simulink model "lab2_next_level"  (R2013a)
settings: Solver=ode1  StartTime=0.0  StopTime=300  FixedStep=0.005  RelTol=1e-3
libraries: simulink x9
Description:
  | Created by MapleSim.
settings Model: ExtModeTrigDuration=10000  Creator=MapleSim  LastModifiedBy=sunnesoft
settings SolverCC: PositivePriorityOrder=on
settings DataIOCC: SignalLoggingSaveFormat=ModelDataLogs  SignalLogging=off  DSMLogging=off
settings OptimizationCC: ExpressionDepthLimit=2147483647  InitFltsAndDblsToZero=on
settings DebuggingCC: SaveWithParameterizedLinksMsg=none  MultiTaskDSMMsg=warning  MultiTaskCondExecSysMsg=none  FcnCallInpInsideContextMsg=UseLocalSettings  StrictBusMsg=None
settings HardwareCC: TargetHWDeviceType=32-bit Generic
settings SFSimCC: SimParseCustomCode=off
settings RTWCC: SystemTargetFile=quarc_win64.tlc  TemplateMakefile=quarc_default_tmf  Description=QUARC Win64 Target  ProcessScript=quarc_win64_make_rtw_hook  IncludeERTFirstTime=on
settings STFCustomTargetCC: TargetPreCompLibLocation=C:\PROGRA~3\QUARC\lib\2011b\win64\release  GeneratePreprocessorConditionals=Disable all  GRTInterface=on  SystemTargetFile=quarc_win64.tlc
settings GRTTargetCC: TargetPreCompLibLocation=C:\PROGRA~3\QUARC\lib\2011b\win64\release  ParMdlRefBuildCompliant=off  CompOptLevelCompliant=off  ConcurrentExecutionCompliant=off  CombineOutputUpdateFcns=off  MatFileLogging=off  GRTInterface=on  ExtMode=on  ExtModeMexFile=quarc_comm

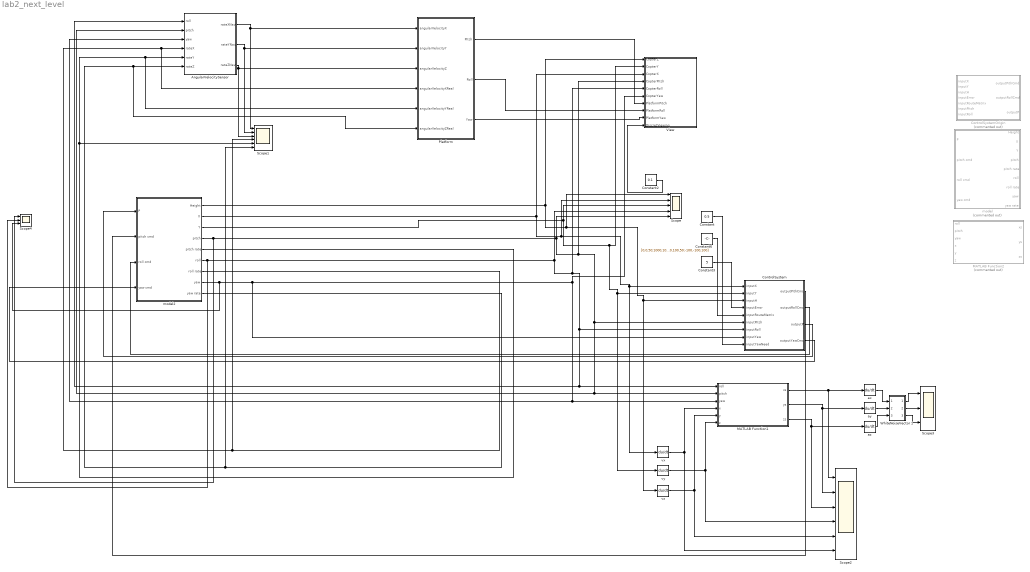
== system lab2_next_level ==
  AngularVelocitySensor : Subsystem
  Constant : Constant  Value=0.5
  Constant2 : Constant  Value=0.1
  Constant3 : Constant  Value=5
  Constant6 : Constant  Value=[0,0,50;1000,1000,50;0,20,50;100,0,50;-30,0,50;100,100,50;-100,-100,100]  VectorParams1D=off
      settings: SamplingMode=Frame based
  ControlSystem : Subsystem
  ControlSystemOrigin : Subsystem  Commented=on
  MATLAB Function1 : MATLAB Function  TreatAsAtomicUnit=on
  MATLAB Function2 : MATLAB Function  Commented=on  TreatAsAtomicUnit=on
  Platform : Subsystem
  Scope : Scope  NumInputPorts=5
      settings: TimeRange=20  YMin=0~0~0~-0.5~-1  YMax=60~450~450~1~0.5
  Scope1 : Scope  NumInputPorts=6
      settings: YMin=-1~-0.00125~-0.00125~-1~-4e-16~-2e-16  YMax=1.25~0.001~0.001~1~4e-16~5e-16
  Scope2 : Scope  NumInputPorts=6
      settings: YMin=-1.38778e-17~-7~0.5~-1~-7~-7  YMax=0.175~-1~3.5~1~-1~-1  SaveName=ScopeData2
  Scope3 : Scope  NumInputPorts=3
      settings: TimeRange=100  YMin=-45~-27.5~-3.5  YMax=15~5~4  SaveName=ScopeData3
  Scope4 : Scope  NumInputPorts=3
      settings: YMin=-0.4~-1~-2e-14  YMax=0.9~1~1e-14  SaveName=ScopeData6
  View : Subsystem
  WhiteNoiseVector 1 : Subsystem
  ax : Derivative
  ay : Derivative
  az : Derivative
  model : Subsystem  Commented=on
  model2 : Subsystem
  vx : Derivative
  vy : Derivative
  vz : Derivative
  wires:
  model2/2("X ") -> View/3(CopterX), ControlSystem/1(inputX), vx/1, Scope/2
  model2/3("Y ") -> View/2(CopterY), ControlSystem/2(inputY), vy/1, Scope/3
  model2/1("Height ") -> View/1(CopterZ), ControlSystem/3(inputH), vz/1, Scope/1
  Constant3/1 -> ControlSystem/4(inputError)
  Constant6/1 -> ControlSystem/5(inputRouteMatrix)
  ControlSystem/1(outputPithCmd) -> model2/2(pitch cmd)
  ControlSystem/2(outputRollCmd) -> model2/3(roll cmd)
  ControlSystem/3(outputP) -> model2/1(P)
  model2/4(pitch) -> Scope4/1, View/4(CopterPitch), ControlSystem/6(inputPitch), AngularVelocitySensor/2(pitch), MATLAB Function1/2(pitch), Scope/5
  model2/8(yaw) -> Scope4/3, ControlSystem/8(inputYaw), View/6(CopterYaw), AngularVelocitySensor/3(yaw), MATLAB Function1/3(yaw)
  vy/1 -> MATLAB Function1/6(z), Scope2/4
  vz/1 -> MATLAB Function1/5(y), Scope2/5
  vx/1 -> MATLAB Function1/4(x), Scope2/6
  MATLAB Function1/1(xs) -> ax/1, Scope2/1
  MATLAB Function1/2(ys) -> ay/1, Scope2/2
  MATLAB Function1/3(zs) -> az/1, Scope2/3
  WhiteNoiseVector 1/1(Out1) -> Scope3/1
  WhiteNoiseVector 1/2(Out2) -> Scope3/2
  WhiteNoiseVector 1/3(Out3) -> Scope3/3
  ay/1 -> WhiteNoiseVector 1/2(In2)
  ax/1 -> WhiteNoiseVector 1/1(In1)
  az/1 -> WhiteNoiseVector 1/3(In3)
  Constant2/1 -> View/10(DiscretViewing)
  model2/5(pitch rate) -> Platform/5(angularVelocityYReal), AngularVelocitySensor/5(rateY), Scope1/5
  model2/9(yaw rate) -> Platform/6(angularVelocityZReal), AngularVelocitySensor/6(rateZ), Scope1/6
  model2/7(roll rate) -> Platform/4(angularVelocityXReal), AngularVelocitySensor/4(rateX), Scope1/4
  AngularVelocitySensor/1(rateXNav) -> Scope1/1, Platform/1(angularVelocityX)
  AngularVelocitySensor/2(rateYNav) -> Platform/2(angularVelocityY), Scope1/2
  AngularVelocitySensor/3(rateZNav) -> Platform/3(angularVelocityZ), Scope1/3
  model2/6(roll) -> Scope4/2, View/5(CopterRoll), ControlSystem/7(inputRoll), AngularVelocitySensor/1(roll), MATLAB Function1/1(roll), Scope/4
  ControlSystem/4(outputYawCmd) -> model2/4(yaw cmd)
  Constant/1 -> ControlSystem/9(inputYawNeed)
  Platform/1(Pitch) -> View/7(PlatformPitch)
  Platform/2(Roll) -> View/8(PlatformRoll)
  Platform/3(Yaw) -> View/9(PlatformYaw)

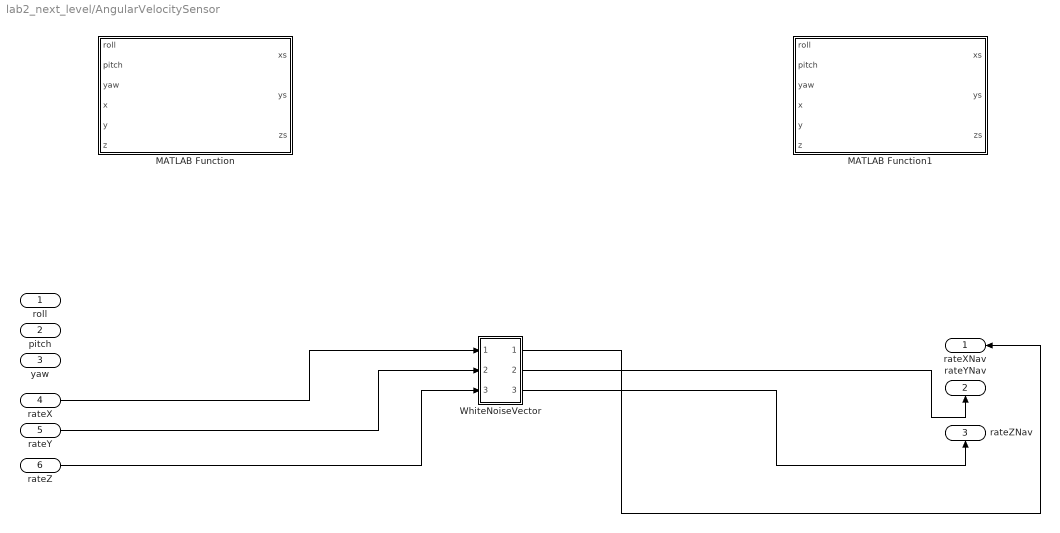
== system lab2_next_level/AngularVelocitySensor ==
  roll : Inport
  pitch : Inport  Port=2
  yaw : Inport  Port=3
  rateX : Inport  Port=4
  rateY : Inport  Port=5
  rateZ : Inport  Port=6
  MATLAB Function : MATLAB Function  TreatAsAtomicUnit=on
  MATLAB Function1 : MATLAB Function  TreatAsAtomicUnit=on
  "WhiteNoiseVector " : Subsystem
  rateXNav : Outport
  rateYNav : Outport  Port=2
  rateZNav : Outport  Port=3
  wires:
  rateX/1 -> "WhiteNoiseVector "/1(In1)
  rateY/1 -> "WhiteNoiseVector "/2(In2)
  rateZ/1 -> "WhiteNoiseVector "/3(In3)
  "WhiteNoiseVector "/1(Out1) -> rateXNav/1
  "WhiteNoiseVector "/2(Out2) -> rateYNav/1
  "WhiteNoiseVector "/3(Out3) -> rateZNav/1

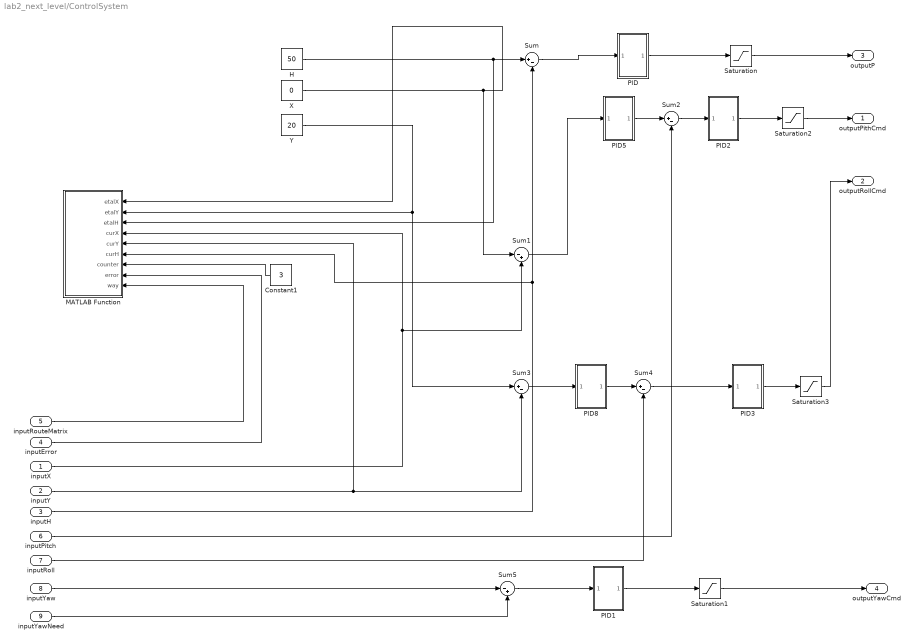
== system lab2_next_level/ControlSystem ==
  inputX : Inport
  inputY : Inport  Port=2
  inputH : Inport  Port=3
  inputError : Inport  Port=4
  inputRouteMatrix : Inport  Port=5
  inputPitch : Inport  Port=6
  inputRoll : Inport  Port=7
  inputYaw : Inport  Port=8
  inputYawNeed : Inport  Port=9
  Constant1 : Constant  InitFcn=|  Value=3
      | coder.extrinsic('set_param');                                    
      | set_param('lab2_next_level/ControlSystem/Constant1','Value','0');
  H : Constant  InitFcn=|  Value=50
      | coder.extrinsic('set_param');                            
      | set_param('lab2_next_level/ControlSystem/H','Value','0');
  MATLAB Function : MATLAB Function  TreatAsAtomicUnit=on
  PID : Subsystem
  PID1 : Subsystem
  PID2 : Subsystem
  PID3 : Subsystem
  PID5 : Subsystem
  PID8 : Subsystem
  Saturation : Saturate  UpperLimit=0.1  LowerLimit=0
  Saturation1 : Saturate  UpperLimit=0.1  LowerLimit=-0.1
  Saturation2 : Saturate  UpperLimit=0.1  LowerLimit=-0.1
  Saturation3 : Saturate  UpperLimit=0.1  LowerLimit=-0.1
  Sum{,2..4} (4 alike) : Sum  Inputs=|+-
  Sum1 : Sum  Inputs=|-+
  Sum5 : Sum  Inputs=|-+
  X : Constant  InitFcn=|  Value=0
      | coder.extrinsic('set_param');                            
      | set_param('lab2_next_level/ControlSystem/X','Value','0');
  Y : Constant  InitFcn=|  Value=20
      | coder.extrinsic('set_param');                            
      | set_param('lab2_next_level/ControlSystem/Y','Value','0');
  outputPithCmd : Outport
  outputRollCmd : Outport  Port=2
  outputP : Outport  Port=3
  outputYawCmd : Outport  Port=4
  wires:
  Saturation2/1 -> outputPithCmd/1
  PID3/1(Out1) -> Saturation3/1
  inputX/1 -> Sum1/2, MATLAB Function/4(curX)
  Saturation3/1 -> outputRollCmd/1
  PID/1(Out1) -> Saturation/1
  Saturation/1 -> outputP/1
  Constant1/1 -> MATLAB Function/7(counter)
  inputPitch/1 -> Sum2/2
  H/1 -> Sum/1, MATLAB Function/3(etalH)
  inputRouteMatrix/1 -> MATLAB Function/9(way)
  inputRoll/1 -> Sum4/2
  Sum3/1 -> PID8/1(In1)
  X/1 -> Sum1/1, MATLAB Function/1(etalX)
  Y/1 -> Sum3/1, MATLAB Function/2(etalY)
  inputError/1 -> MATLAB Function/8(error)
  inputY/1 -> Sum3/2, MATLAB Function/5(curY)
  Sum/1 -> PID/1(In1)
  inputH/1 -> MATLAB Function/6(curH), Sum/2
  PID2/1(Out1) -> Saturation2/1
  Sum1/1 -> PID5/1(In1)
  Sum2/1 -> PID2/1(In1)
  Sum4/1 -> PID3/1(In1)
  PID5/1(Out1) -> Sum2/1
  PID8/1(Out1) -> Sum4/1
  Saturation1/1 -> outputYawCmd/1
  PID1/1(Out1) -> Saturation1/1
  inputYaw/1 -> Sum5/1
  inputYawNeed/1 -> Sum5/2
  Sum5/1 -> PID1/1(In1)

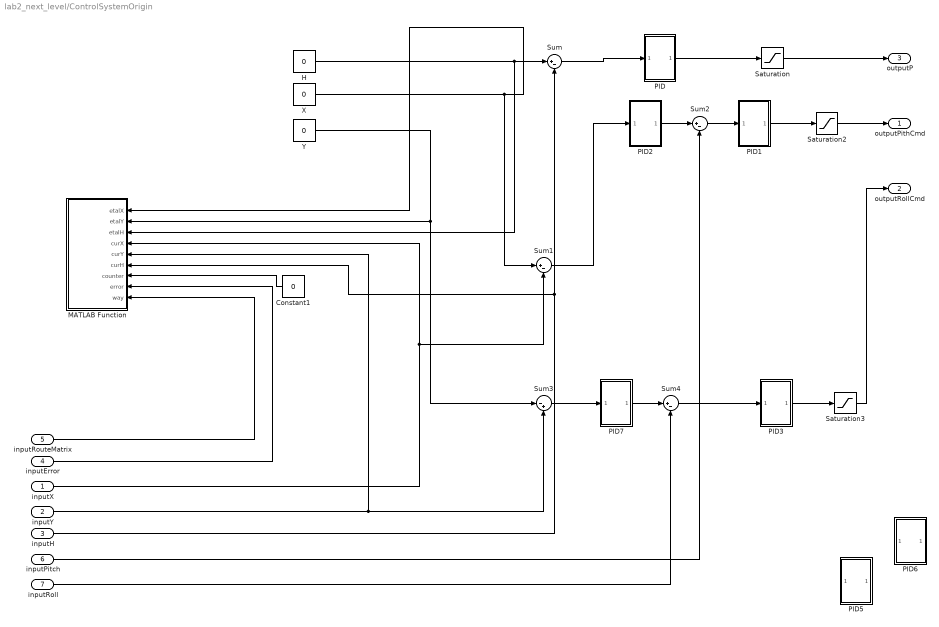
== system lab2_next_level/ControlSystemOrigin ==
  inputX : Inport
  inputY : Inport  Port=2
  inputH : Inport  Port=3
  inputError : Inport  Port=4
  inputRouteMatrix : Inport  Port=5
  inputPitch : Inport  Port=6
  inputRoll : Inport  Port=7
  Constant1 : Constant  InitFcn=|  Value=0
      | coder.extrinsic('set_param');                                    
      | set_param('lab2_next_level/ControlSystem/Constant1','Value','0');
  H : Constant  InitFcn=|  Value=0
      | coder.extrinsic('set_param');                            
      | set_param('lab2_next_level/ControlSystem/H','Value','0');
  MATLAB Function : MATLAB Function  TreatAsAtomicUnit=on
  PID : Subsystem
  PID1 : Subsystem
  PID2 : Subsystem
  PID3 : Subsystem
  PID5 : Subsystem
  PID6 : Subsystem
  PID7 : Subsystem
  Saturation : Saturate  UpperLimit=0.1  LowerLimit=0
  Saturation2 : Saturate  UpperLimit=0.1  LowerLimit=-0.1
  Saturation3 : Saturate  UpperLimit=0.01  LowerLimit=-0.01
  Sum{,1..2,4} (4 alike) : Sum  Inputs=|+-
  Sum3 : Sum  Inputs=|-+
  X : Constant  InitFcn=|  Value=0
      | coder.extrinsic('set_param');                            
      | set_param('lab2_next_level/ControlSystem/X','Value','0');
  Y : Constant  InitFcn=|  Value=0
      | coder.extrinsic('set_param');                            
      | set_param('lab2_next_level/ControlSystem/Y','Value','0');
  outputPithCmd : Outport
  outputRollCmd : Outport  Port=2
  outputP : Outport  Port=3
  wires:
  Saturation2/1 -> outputPithCmd/1
  PID3/1(Out1) -> Saturation3/1
  inputX/1 -> Sum1/2, MATLAB Function/4(curX)
  Saturation3/1 -> outputRollCmd/1
  PID/1(Out1) -> Saturation/1
  Saturation/1 -> outputP/1
  Constant1/1 -> MATLAB Function/7(counter)
  inputPitch/1 -> Sum2/2
  H/1 -> Sum/1, MATLAB Function/3(etalH)
  inputRouteMatrix/1 -> MATLAB Function/9(way)
  inputRoll/1 -> Sum4/2
  Sum3/1 -> PID7/1(In1)
  X/1 -> Sum1/1, MATLAB Function/1(etalX)
  Y/1 -> Sum3/1, MATLAB Function/2(etalY)
  inputError/1 -> MATLAB Function/8(error)
  inputY/1 -> Sum3/2, MATLAB Function/5(curY)
  Sum/1 -> PID/1(In1)
  inputH/1 -> MATLAB Function/6(curH), Sum/2
  PID1/1(Out1) -> Saturation2/1
  Sum1/1 -> PID2/1(In1)
  Sum2/1 -> PID1/1(In1)
  Sum4/1 -> PID3/1(In1)
  PID2/1(Out1) -> Sum2/1
  PID7/1(Out1) -> Sum4/1

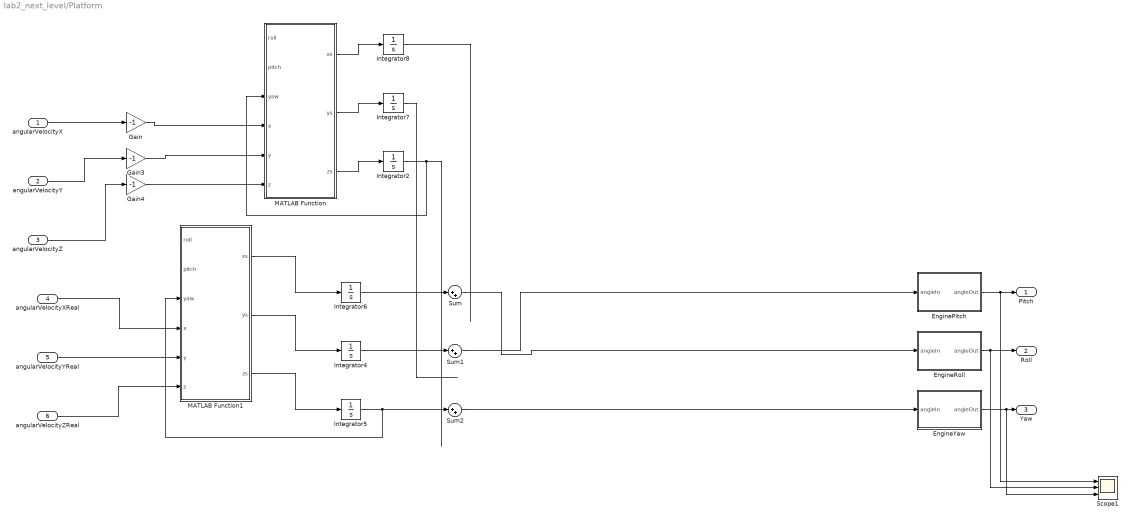
== system lab2_next_level/Platform ==
  angularVelocityX : Inport
  angularVelocityY : Inport  Port=2
  angularVelocityZ : Inport  Port=3
  angularVelocityXReal : Inport  Port=4
  angularVelocityYReal : Inport  Port=5
  angularVelocityZReal : Inport  Port=6
  EnginePitch : Subsystem
  EngineRoll : Subsystem
  EngineYaw : Subsystem
  Gain : Gain  Gain=-1
  Gain3 : Gain  Gain=-1
  Gain4 : Gain  Gain=-1
  Integrator{2,4..8} (6 alike) : Integrator  LimitOutput=on  UpperSaturationLimit=1  LowerSaturationLimit=-1
  MATLAB Function : MATLAB Function  TreatAsAtomicUnit=on
  MATLAB Function1 : MATLAB Function  TreatAsAtomicUnit=on
  Scope1 : Scope  NumInputPorts=3
      settings: TimeRange=10  YMin=-0.002~-0.0007~-0.0025  YMax=0.004~0.0003~0.0025  SaveName=ScopeData4
  Sum : Sum  Inputs=|++
  Sum1 : Sum  Inputs=|++
  Sum2 : Sum  Inputs=|++
  Pitch : Outport
  Roll : Outport  Port=2
  Yaw : Outport  Port=3
  wires:
  Integrator7/1 -> ?
  Integrator2/1 -> MATLAB Function/3(yaw)
  MATLAB Function/3(zs) -> Integrator2/1
  Integrator8/1 -> ?
  MATLAB Function/1(xs) -> Integrator8/1
  MATLAB Function/2(ys) -> Integrator7/1
  Gain/1 -> MATLAB Function/4(x)
  Gain3/1 -> MATLAB Function/5(y)
  Gain4/1 -> MATLAB Function/6(z)
  Integrator6/1 -> Sum/1
  Integrator4/1 -> Sum1/1
  Integrator5/1 -> MATLAB Function1/3(yaw), Sum2/1
  Sum2/1 -> EngineYaw/1(angleIn)
  Sum/1 -> EngineRoll/1(angleIn)
  Sum1/1 -> EnginePitch/1(angleIn)
  MATLAB Function1/1(xs) -> Integrator6/1
  MATLAB Function1/2(ys) -> Integrator4/1
  MATLAB Function1/3(zs) -> Integrator5/1
  angularVelocityX/1 -> Gain/1
  angularVelocityY/1 -> Gain3/1
  angularVelocityZ/1 -> Gain4/1
  angularVelocityXReal/1 -> MATLAB Function1/4(x)
  angularVelocityYReal/1 -> MATLAB Function1/5(y)
  angularVelocityZReal/1 -> MATLAB Function1/6(z)
  EngineRoll/1(angleOut) -> Scope1/2, Roll/1
  EngineYaw/1(angleOut) -> Scope1/3, Yaw/1
  EnginePitch/1(angleOut) -> Scope1/1, Pitch/1

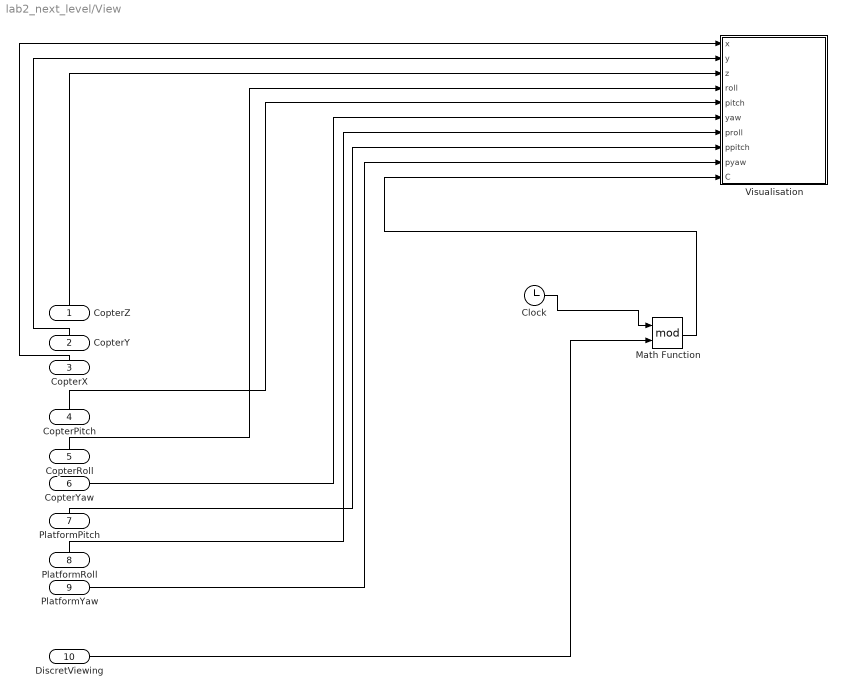
== system lab2_next_level/View ==
  CopterZ : Inport
  CopterY : Inport  Port=2
  CopterX : Inport  Port=3
  CopterPitch : Inport  Port=4
  CopterRoll : Inport  Port=5
  CopterYaw : Inport  Port=6
  PlatformPitch : Inport  Port=7
  PlatformRoll : Inport  Port=8
  PlatformYaw : Inport  Port=9
  DiscretViewing : Inport  Port=10
  Clock : Clock
  Math Function : Math  Operator=mod  SaturateOnIntegerOverflow=on
  Visualisation : MATLAB Function  TreatAsAtomicUnit=on
  wires:
  DiscretViewing/1 -> Math Function/2
  Math Function/1 -> Visualisation/10(C)
  Clock/1 -> Math Function/1
  CopterYaw/1 -> Visualisation/6(yaw)
  CopterZ/1 -> Visualisation/3(z)
  CopterPitch/1 -> Visualisation/5(pitch)
  CopterRoll/1 -> Visualisation/4(roll)
  CopterY/1 -> Visualisation/2(y)
  CopterX/1 -> Visualisation/1(x)
  PlatformYaw/1 -> Visualisation/9(pyaw)
  PlatformPitch/1 -> Visualisation/8(ppitch)
  PlatformRoll/1 -> Visualisation/7(proll)

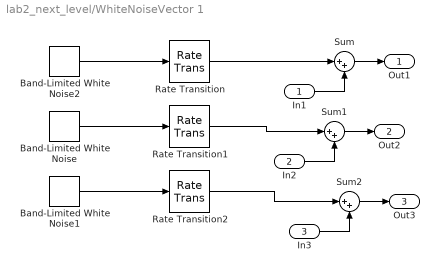
== system lab2_next_level/WhiteNoiseVector 1 ==
  In1 : Inport
  In2 : Inport  Port=2
  In3 : Inport  Port=3
  Band-Limited White Noise : simulink/Sources/Band-Limited White Noise  Cov=[0.1]  Ts=0.1  seed=[23341]
  Band-Limited White Noise1 : simulink/Sources/Band-Limited White Noise  Cov=[0.1]  Ts=0.1  seed=[23341]
  Band-Limited White Noise2 : simulink/Sources/Band-Limited White Noise  Cov=[0.1]  Ts=0.1  seed=[23341]
  Rate Transition : RateTransition
  Rate Transition1 : RateTransition
  Rate Transition2 : RateTransition
  Sum : Sum  Inputs=|++
  Sum1 : Sum  Inputs=|++
  Sum2 : Sum  Inputs=|++
  Out1 : Outport
  Out2 : Outport  Port=2
  Out3 : Outport  Port=3
  wires:
  Band-Limited White Noise2/1 -> Rate Transition/1
  Band-Limited White Noise/1 -> Rate Transition1/1
  Sum/1 -> Out1/1
  Band-Limited White Noise1/1 -> Rate Transition2/1
  Rate Transition/1 -> Sum/1
  In1/1 -> Sum/2
  Sum1/1 -> Out2/1
  Rate Transition1/1 -> Sum1/1
  In2/1 -> Sum1/2
  Sum2/1 -> Out3/1
  Rate Transition2/1 -> Sum2/1
  In3/1 -> Sum2/2

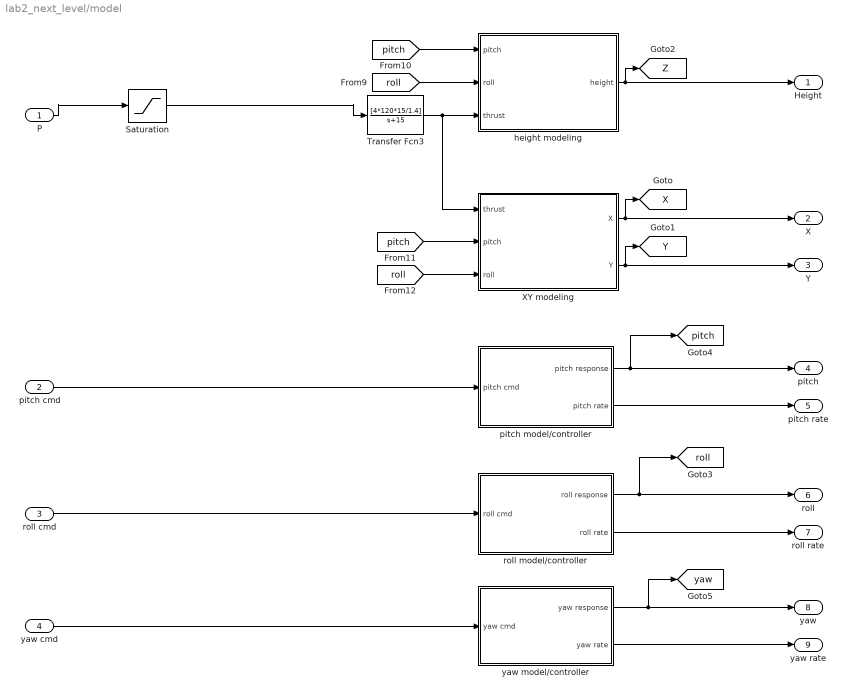
== system lab2_next_level/model ==
  P : Inport
  pitch cmd : Inport  Port=2
  roll cmd : Inport  Port=3
  yaw cmd : Inport  Port=4
  Saturation : Saturate  UpperLimit=0.1  LowerLimit=0
  Transfer Fcn3 : TransferFcn  Numerator=[4*120*15/1.4]  Denominator=[1 15]
  XY modeling : Subsystem
  height modeling : Subsystem
  pitch model/controller : Subsystem
  roll model/controller : Subsystem
  yaw model/controller : Subsystem
  "Height " : Outport
  "X " : Outport  Port=2
  "Y " : Outport  Port=3
  pitch : Outport  Port=4
  pitch rate : Outport  Port=5
  roll : Outport  Port=6
  roll rate : Outport  Port=7
  yaw : Outport  Port=8
  yaw rate : Outport  Port=9
  tag scope: X=global, Y=global, Z=global, pitch=global, roll=global, yaw=global
  wires:
  yaw cmd/1 -> yaw model/controller/1(yaw cmd)
  roll cmd/1 -> roll model/controller/1(roll cmd)
  pitch cmd/1 -> pitch model/controller/1(pitch cmd)
  P/1 -> Saturation/1
  yaw model/controller/2(yaw rate) -> yaw rate/1
  roll model/controller/2(roll rate) -> roll rate/1
  pitch model/controller/2(pitch rate) -> pitch rate/1
  XY modeling/2(Y) -> "Y "/1, [Y]
  XY modeling/1(X) -> "X "/1, [X]
  [roll] -> XY modeling/3(roll)
  [pitch] -> XY modeling/2(pitch)
  Transfer Fcn3/1 -> XY modeling/1(thrust), height modeling/3(thrust)
  [roll] -> height modeling/2(roll)
  [pitch] -> height modeling/1(pitch)
  height modeling/1(height) -> "Height "/1, [Z]
  yaw model/controller/1(yaw response) -> yaw/1, [yaw]
  roll model/controller/1(roll response) -> roll/1, [roll]
  pitch model/controller/1(pitch response) -> [pitch], pitch/1
  Saturation/1 -> Transfer Fcn3/1

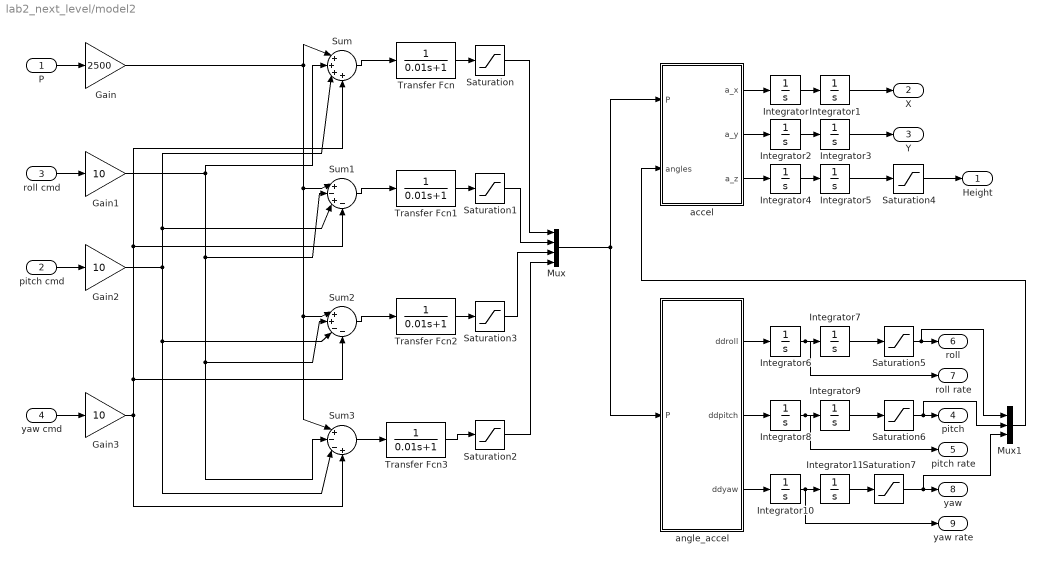
== system lab2_next_level/model2 ==
  P : Inport
  pitch cmd : Inport  Port=2
  roll cmd : Inport  Port=3
  yaw cmd : Inport  Port=4
  Gain : Gain  Gain=2500
  Gain1 : Gain  Gain=10
  Gain2 : Gain  Gain=10
  Gain3 : Gain  Gain=10
  Integrator{,1..5,10..11} (8 alike) : Integrator
  Integrator{6..9} (4 alike) : Integrator  LimitOutput=on  UpperSaturationLimit=1  LowerSaturationLimit=-1
  Mux : Mux
  Mux1 : Mux  Inputs=3
  Saturation{,1..3} (4 alike) : Saturate  UpperLimit=500  LowerLimit=0
  Saturation4 : Saturate  UpperLimit=100000000  LowerLimit=0
  Saturation5 : Saturate  UpperLimit=1  LowerLimit=-1
  Saturation6 : Saturate  UpperLimit=1  LowerLimit=-1
  Saturation7 : Saturate  UpperLimit=1  LowerLimit=-1
  Sum : Sum  Inputs=|++++
  Sum1 : Sum  Inputs=|+-+-
  Sum2 : Sum  Inputs=|++--
  Sum3 : Sum  Inputs=|+--+
  Transfer Fcn{,1..3} (4 alike) : TransferFcn  Denominator=[0.01 1]
  accel : MATLAB Function  TreatAsAtomicUnit=on
  angle_accel : MATLAB Function  TreatAsAtomicUnit=on
  "Height " : Outport
  "X " : Outport  Port=2
  "Y " : Outport  Port=3
  pitch : Outport  Port=4
  pitch rate : Outport  Port=5
  roll : Outport  Port=6
  roll rate : Outport  Port=7
  yaw : Outport  Port=8
  yaw rate : Outport  Port=9
  wires:
  P/1 -> Gain/1
  Gain/1 -> Sum1/1, Sum3/1, Sum2/1, Sum/1
  Sum/1 -> Transfer Fcn/1
  Sum1/1 -> Transfer Fcn1/1
  Sum2/1 -> Transfer Fcn2/1
  Sum3/1 -> Transfer Fcn3/1
  Transfer Fcn/1 -> Saturation/1
  Mux/1 -> accel/1(P), angle_accel/1(P)
  Integrator/1 -> Integrator1/1
  Integrator2/1 -> Integrator3/1
  Integrator4/1 -> Integrator5/1
  accel/1(a_x) -> Integrator/1
  accel/2(a_y) -> Integrator2/1
  accel/3(a_z) -> Integrator4/1
  Integrator1/1 -> "X "/1
  Integrator3/1 -> "Y "/1
  Integrator5/1 -> Saturation4/1
  angle_accel/1(ddroll) -> Integrator6/1
  Integrator6/1 -> roll rate/1, Integrator7/1
  angle_accel/3(ddyaw) -> Integrator10/1
  angle_accel/2(ddpitch) -> Integrator8/1
  Integrator8/1 -> pitch rate/1, Integrator9/1
  Integrator10/1 -> yaw rate/1, Integrator11/1
  Integrator7/1 -> Saturation5/1
  Integrator9/1 -> Saturation6/1
  Integrator11/1 -> Saturation7/1
  Saturation/1 -> Mux/1
  Transfer Fcn1/1 -> Saturation1/1
  Saturation1/1 -> Mux/2
  Saturation2/1 -> Mux/4
  Transfer Fcn2/1 -> Saturation3/1
  Saturation3/1 -> Mux/3
  yaw cmd/1 -> Gain3/1
  Saturation4/1 -> "Height "/1
  Saturation5/1 -> Mux1/1, roll/1
  Saturation6/1 -> Mux1/2, pitch/1
  roll cmd/1 -> Gain1/1
  pitch cmd/1 -> Gain2/1
  Saturation7/1 -> Mux1/3, yaw/1
  Mux1/1 -> accel/2(angles)
  Gain1/1 -> Sum2/2, Sum3/2, Sum1/2, Sum/2
  Gain2/1 -> Sum1/3, Sum/3, Sum2/3, Sum3/3
  Gain3/1 -> Sum2/4, Sum1/4, Sum/4, Sum3/4
  Transfer Fcn3/1 -> Saturation2/1

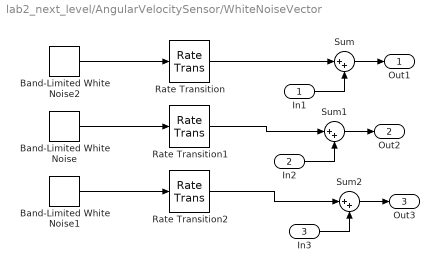
== system lab2_next_level/AngularVelocitySensor/WhiteNoiseVector  ==
  In1 : Inport
  In2 : Inport  Port=2
  In3 : Inport  Port=3
  Band-Limited White Noise : simulink/Sources/Band-Limited White Noise  Cov=[1e-8]  Ts=0.1  seed=[23341]
  Band-Limited White Noise1 : simulink/Sources/Band-Limited White Noise  Cov=[1e-8]  Ts=0.1  seed=[23341]
  Band-Limited White Noise2 : simulink/Sources/Band-Limited White Noise  Cov=[1e-8]  Ts=0.1  seed=[23341]
  Rate Transition : RateTransition
  Rate Transition1 : RateTransition
  Rate Transition2 : RateTransition
  Sum : Sum  Inputs=|++
  Sum1 : Sum  Inputs=|++
  Sum2 : Sum  Inputs=|++
  Out1 : Outport
  Out2 : Outport  Port=2
  Out3 : Outport  Port=3
  wires:
  Band-Limited White Noise2/1 -> Rate Transition/1
  Band-Limited White Noise/1 -> Rate Transition1/1
  Sum/1 -> Out1/1
  Band-Limited White Noise1/1 -> Rate Transition2/1
  Rate Transition/1 -> Sum/1
  In1/1 -> Sum/2
  Sum1/1 -> Out2/1
  Rate Transition1/1 -> Sum1/1
  In2/1 -> Sum1/2
  Sum2/1 -> Out3/1
  Rate Transition2/1 -> Sum2/1
  In3/1 -> Sum2/2

== system lab2_next_level/ControlSystem/PID ==
  In1 : Inport
  Derivative : Derivative
  Gain : Gain  Gain=0.007
  Gain1 : Gain  Gain=0.0006
  Gain2 : Gain  Gain=0.02
  Gain3 : Gain
  Integrator : Integrator
  Sum1 : Sum  Inputs=|+++
  Out1 : Outport
  wires:
  Gain1/1 -> Integrator/1
  Gain3/1 -> Sum1/1
  Integrator/1 -> Sum1/2
  Gain/1 -> Gain3/1
  In1/1 -> Gain1/1, Gain/1, Gain2/1
  Derivative/1 -> Sum1/3
  Gain2/1 -> Derivative/1
  Sum1/1 -> Out1/1

== system lab2_next_level/ControlSystem/PID1 ==
  In1 : Inport
  Derivative : Derivative
  Gain : Gain  Gain=0.012
  Gain1 : Gain  Gain=0.00048
  Gain2 : Gain  Gain=0.075
  Gain3 : Gain
  Integrator : Integrator
  Sum1 : Sum  Inputs=|+++
  Out1 : Outport
  wires:
  Gain1/1 -> Integrator/1
  Gain3/1 -> Sum1/1
  Integrator/1 -> Sum1/2
  Gain/1 -> Gain3/1
  In1/1 -> Gain1/1, Gain/1, Gain2/1
  Derivative/1 -> Sum1/3
  Gain2/1 -> Derivative/1
  Sum1/1 -> Out1/1

== system lab2_next_level/ControlSystem/PID2 ==
  In1 : Inport
  Derivative : Derivative
  Gain : Gain  Gain=0.02
  Gain1 : Gain  Gain=1e-9
  Gain2 : Gain  Gain=0.2
  Gain3 : Gain
  Integrator : Integrator
  Sum1 : Sum  Inputs=|+++
  Out1 : Outport
  wires:
  Gain1/1 -> Integrator/1
  Gain3/1 -> Sum1/1
  Integrator/1 -> Sum1/2
  Gain/1 -> Gain3/1
  In1/1 -> Gain1/1, Gain/1, Gain2/1
  Derivative/1 -> Sum1/3
  Gain2/1 -> Derivative/1
  Sum1/1 -> Out1/1

== system lab2_next_level/ControlSystem/PID3 ==
  In1 : Inport
  Derivative : Derivative
  Gain : Gain  Gain=0.02
  Gain1 : Gain  Gain=1e-9
  Gain2 : Gain  Gain=0.2
  Gain3 : Gain
  Integrator : Integrator
  Sum1 : Sum  Inputs=|+++
  Out1 : Outport
  wires:
  Gain1/1 -> Integrator/1
  Gain3/1 -> Sum1/1
  Integrator/1 -> Sum1/2
  Gain/1 -> Gain3/1
  In1/1 -> Gain1/1, Gain/1, Gain2/1
  Derivative/1 -> Sum1/3
  Gain2/1 -> Derivative/1
  Sum1/1 -> Out1/1

== system lab2_next_level/ControlSystem/PID5 ==
  In1 : Inport
  Derivative : Derivative
  Gain : Gain  Gain=0.1
  Gain1 : Gain  Gain=1e-9
  Gain2 : Gain  Gain=0.35
  Gain3 : Gain
  Integrator : Integrator
  Sum1 : Sum  Inputs=|+++
  Out1 : Outport
  wires:
  Gain1/1 -> Integrator/1
  Gain3/1 -> Sum1/1
  Integrator/1 -> Sum1/2
  Gain/1 -> Gain3/1
  In1/1 -> Gain1/1, Gain/1, Gain2/1
  Derivative/1 -> Sum1/3
  Gain2/1 -> Derivative/1
  Sum1/1 -> Out1/1

== system lab2_next_level/ControlSystem/PID8 ==
  In1 : Inport
  Derivative : Derivative
  Gain : Gain  Gain=0.1
  Gain1 : Gain  Gain=1e-9
  Gain2 : Gain  Gain=0.35
  Gain3 : Gain
  Integrator : Integrator
  Sum1 : Sum  Inputs=|+++
  Out1 : Outport
  wires:
  Gain1/1 -> Integrator/1
  Gain3/1 -> Sum1/1
  Integrator/1 -> Sum1/2
  Gain/1 -> Gain3/1
  In1/1 -> Gain1/1, Gain/1, Gain2/1
  Derivative/1 -> Sum1/3
  Gain2/1 -> Derivative/1
  Sum1/1 -> Out1/1

== system lab2_next_level/ControlSystemOrigin/PID ==
  In1 : Inport
  Derivative : Derivative
  Gain : Gain  Gain=0.006
  Gain1 : Gain  Gain=3.831578947e-04
  Gain2 : Gain  Gain=0.0361325
  Gain3 : Gain
  Integrator : Integrator
  Sum1 : Sum  Inputs=|+++
  Out1 : Outport
  wires:
  Gain1/1 -> Integrator/1
  Gain3/1 -> Sum1/1
  Integrator/1 -> Sum1/2
  Gain/1 -> Gain3/1
  In1/1 -> Gain1/1, Gain/1, Gain2/1
  Derivative/1 -> Sum1/3
  Gain2/1 -> Derivative/1
  Sum1/1 -> Out1/1

== system lab2_next_level/ControlSystemOrigin/PID1 ==
  In1 : Inport
  Derivative : Derivative
  Gain : Gain  Gain=6e-03
  Gain1 : Gain  Gain=6e-9
  Gain2 : Gain  Gain=0.0255
  Gain3 : Gain
  Integrator : Integrator
  Sum1 : Sum  Inputs=|+++
  Out1 : Outport
  wires:
  Gain1/1 -> Integrator/1
  Gain3/1 -> Sum1/1
  Integrator/1 -> Sum1/2
  Gain/1 -> Gain3/1
  In1/1 -> Gain1/1, Gain/1, Gain2/1
  Derivative/1 -> Sum1/3
  Gain2/1 -> Derivative/1
  Sum1/1 -> Out1/1

== system lab2_next_level/ControlSystemOrigin/PID2 ==
  In1 : Inport
  Derivative : Derivative
  Gain : Gain  Gain=0.010
  Gain1 : Gain  Gain=7.058823529e-09
  Gain2 : Gain  Gain=0.141875
  Gain3 : Gain
  Integrator : Integrator
  Sum1 : Sum  Inputs=|+++
  Out1 : Outport
  wires:
  Gain1/1 -> Integrator/1
  Gain3/1 -> Sum1/1
  Integrator/1 -> Sum1/2
  Gain/1 -> Gain3/1
  In1/1 -> Gain1/1, Gain/1, Gain2/1
  Derivative/1 -> Sum1/3
  Gain2/1 -> Derivative/1
  Sum1/1 -> Out1/1

== system lab2_next_level/ControlSystemOrigin/PID3 ==
  In1 : Inport
  Derivative : Derivative
  Gain : Gain  Gain=5e-03
  Gain1 : Gain  Gain=6e-9
  Gain2 : Gain  Gain=0.035
  Gain3 : Gain
  Integrator : Integrator
  Sum1 : Sum  Inputs=|+++
  Out1 : Outport
  wires:
  Gain1/1 -> Integrator/1
  Gain3/1 -> Sum1/1
  Integrator/1 -> Sum1/2
  Gain/1 -> Gain3/1
  In1/1 -> Gain1/1, Gain/1, Gain2/1
  Derivative/1 -> Sum1/3
  Gain2/1 -> Derivative/1
  Sum1/1 -> Out1/1

== system lab2_next_level/ControlSystemOrigin/PID5 ==
  In1 : Inport
  Derivative : Derivative
  Gain : Gain  Gain=0.0005
  Gain1 : Gain  Gain=2e-09
  Gain2 : Gain  Gain=0.0545
  Gain3 : Gain
  Integrator : Integrator
  Sum1 : Sum  Inputs=|+++
  Out1 : Outport
  wires:
  Gain1/1 -> Integrator/1
  Gain3/1 -> Sum1/1
  Integrator/1 -> Sum1/2
  Gain/1 -> Gain3/1
  In1/1 -> Gain1/1, Gain/1, Gain2/1
  Derivative/1 -> Sum1/3
  Gain2/1 -> Derivative/1
  Sum1/1 -> Out1/1

== system lab2_next_level/ControlSystemOrigin/PID6 ==
  In1 : Inport
  Derivative : Derivative
  Gain : Gain  Gain=1e-03
  Gain1 : Gain  Gain=2.4e-07
  Gain2 : Gain  Gain=9e-05
  Gain3 : Gain
  Integrator : Integrator
  Sum1 : Sum  Inputs=|+++
  Out1 : Outport
  wires:
  Gain1/1 -> Integrator/1
  Gain3/1 -> Sum1/1
  Integrator/1 -> Sum1/2
  Gain/1 -> Gain3/1
  In1/1 -> Gain1/1, Gain2/1, Gain/1
  Derivative/1 -> Sum1/3
  Gain2/1 -> Derivative/1
  Sum1/1 -> Out1/1

== system lab2_next_level/ControlSystemOrigin/PID7 ==
  In1 : Inport
  Derivative : Derivative
  Gain : Gain  Gain=0.013
  Gain1 : Gain  Gain=7.058823529e-08
  Gain2 : Gain  Gain=0.171875
  Gain3 : Gain
  Integrator : Integrator
  Sum1 : Sum  Inputs=|+++
  Out1 : Outport
  wires:
  Gain1/1 -> Integrator/1
  Gain3/1 -> Sum1/1
  Integrator/1 -> Sum1/2
  Gain/1 -> Gain3/1
  In1/1 -> Gain1/1, Gain/1, Gain2/1
  Derivative/1 -> Sum1/3
  Gain2/1 -> Derivative/1
  Sum1/1 -> Out1/1

== system lab2_next_level/Platform/EnginePitch ==
  angleIn : Inport
  Band-Limited White Noise2 : simulink/Sources/Band-Limited White Noise  Cov=[0.00001]  Ts=0.1  seed=[23341]
  Gain : Gain  Gain=10
  Integrator1 : Integrator
  PID2 : Subsystem
  Rate Transition : RateTransition
  Saturation : Saturate
  Saturation1 : Saturate  UpperLimit=1  LowerLimit=-1
  Sum : Sum  Inputs=|+-
  Sum2 : Sum  Inputs=|++
  Transfer Fcn : TransferFcn  Denominator=[1 1]
  angleOut : Outport
  wires:
  PID2/1(Out1) -> Saturation1/1
  Gain/1 -> Transfer Fcn/1
  Rate Transition/1 -> Sum2/2
  Band-Limited White Noise2/1 -> Rate Transition/1
  Transfer Fcn/1 -> Sum2/1
  Sum2/1 -> Integrator1/1
  Integrator1/1 -> angleOut/1, Sum/2
  Sum/1 -> PID2/1(In1)
  angleIn/1 -> Saturation/1
  Saturation/1 -> Sum/1
  Saturation1/1 -> Gain/1

== system lab2_next_level/Platform/EngineRoll ==
  angleIn : Inport
  Band-Limited White Noise2 : simulink/Sources/Band-Limited White Noise  Cov=[0.00001]  Ts=0.1  seed=[23341]
  Gain : Gain  Gain=100
  Integrator1 : Integrator
  PID2 : Subsystem
  Rate Transition : RateTransition
  Saturation : Saturate  UpperLimit=1  LowerLimit=-1
  Saturation1 : Saturate  UpperLimit=1  LowerLimit=-1
  Sum : Sum  Inputs=|+-
  Sum2 : Sum  Inputs=|++
  Transfer Fcn : TransferFcn  Denominator=[1 1]
  angleOut : Outport
  wires:
  PID2/1(Out1) -> Saturation1/1
  Gain/1 -> Transfer Fcn/1
  Rate Transition/1 -> Sum2/2
  Band-Limited White Noise2/1 -> Rate Transition/1
  Transfer Fcn/1 -> Sum2/1
  Sum2/1 -> Integrator1/1
  Integrator1/1 -> angleOut/1, Sum/2
  Sum/1 -> PID2/1(In1)
  angleIn/1 -> Saturation/1
  Saturation/1 -> Sum/1
  Saturation1/1 -> Gain/1

== system lab2_next_level/Platform/EngineYaw ==
  angleIn : Inport
  Band-Limited White Noise2 : simulink/Sources/Band-Limited White Noise  Cov=[0.00001]  Ts=0.1  seed=[23341]
  Gain : Gain  Gain=10
  Integrator1 : Integrator
  PID2 : Subsystem
  Rate Transition : RateTransition
  Saturation : Saturate
  Saturation1 : Saturate  UpperLimit=1  LowerLimit=-1
  Sum : Sum  Inputs=|+-
  Sum2 : Sum  Inputs=|++
  Transfer Fcn : TransferFcn  Denominator=[1 1]
  angleOut : Outport
  wires:
  PID2/1(Out1) -> Saturation1/1
  Gain/1 -> Transfer Fcn/1
  Rate Transition/1 -> Sum2/2
  Band-Limited White Noise2/1 -> Rate Transition/1
  Transfer Fcn/1 -> Sum2/1
  Sum2/1 -> Integrator1/1
  Integrator1/1 -> angleOut/1, Sum/2
  Sum/1 -> PID2/1(In1)
  angleIn/1 -> Saturation/1
  Saturation/1 -> Sum/1
  Saturation1/1 -> Gain/1

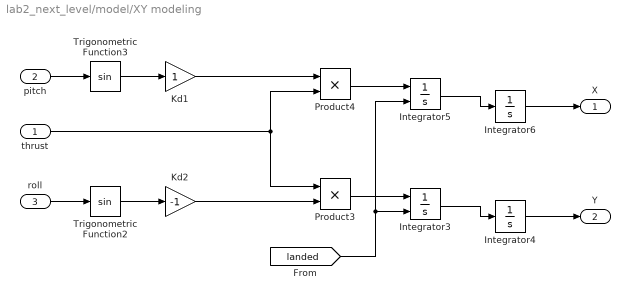
== system lab2_next_level/model/XY modeling ==
  thrust : Inport
  pitch : Inport  Port=2
  roll : Inport  Port=3
  Integrator3 : Integrator  ExternalReset=level
  Integrator4 : Integrator  LowerSaturationLimit=-0.5
  Integrator5 : Integrator  ExternalReset=level
  Integrator6 : Integrator  LowerSaturationLimit=-0.5
  Kd1 : Gain
  Kd2 : Gain  Gain=-1
  Product3 : Product  RndMeth=Zero
  Product4 : Product  RndMeth=Zero
  Trigonometric Function2 : Trigonometry
  Trigonometric Function3 : Trigonometry
  X : Outport
  Y : Outport  Port=2
  wires:
  Trigonometric Function2/1 -> Kd2/1
  Product3/1 -> Integrator3/1
  Integrator3/1 -> Integrator4/1
  Product4/1 -> Integrator5/1
  Integrator5/1 -> Integrator6/1
  Trigonometric Function3/1 -> Kd1/1
  Kd1/1 -> Product4/1
  Kd2/1 -> Product3/2
  pitch/1 -> Trigonometric Function3/1
  thrust/1 -> Product3/1, Product4/2
  roll/1 -> Trigonometric Function2/1
  Integrator4/1 -> Y/1
  Integrator6/1 -> X/1
  [landed] -> Integrator5/2, Integrator3/2

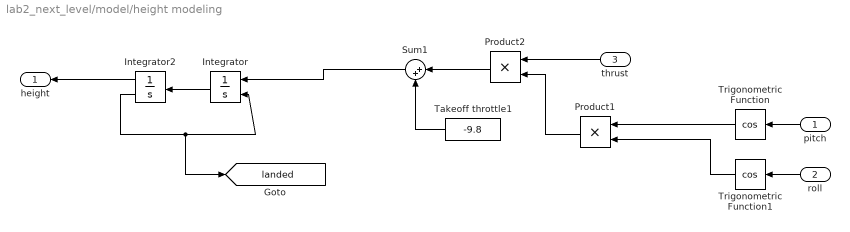
== system lab2_next_level/model/height modeling ==
  pitch : Inport
  roll : Inport  Port=2
  thrust : Inport  Port=3
  Integrator : Integrator  ExternalReset=falling
  Integrator2 : Integrator  InitialCondition=0.236  LimitOutput=on  LowerSaturationLimit=0.236  ShowSaturationPort=on
  Product1 : Product  RndMeth=Zero
  Product2 : Product  RndMeth=Zero
  Sum1 : Sum  Inputs=|++
  Takeoff throttle1 : Constant  Value=-9.8
  Trigonometric Function : Trigonometry  Operator=cos
  Trigonometric Function1 : Trigonometry  Operator=cos
  height : Outport
  tag scope: landed=global
  wires:
  Trigonometric Function/1 -> Product1/1
  Trigonometric Function1/1 -> Product1/2
  Product2/1 -> Sum1/1
  Product1/1 -> Product2/2
  Sum1/1 -> Integrator/1
  Takeoff throttle1/1 -> Sum1/2
  Integrator2/1 -> height/1
  Integrator/1 -> Integrator2/1
  thrust/1 -> Product2/1
  pitch/1 -> Trigonometric Function/1
  roll/1 -> Trigonometric Function1/1
  Integrator2/2 -> Integrator/2, [landed]

== system lab2_next_level/model/pitch model//controller ==
  pitch cmd : Inport
  pitch model : Subsystem
  pitch response : Outport
  pitch rate : Outport  Port=2
  wires:
  pitch model/2(pitch rate) -> pitch rate/1
  pitch cmd/1 -> pitch model/1(u_pitch)
  pitch model/1(pitch) -> pitch response/1

== system lab2_next_level/model/roll model//controller ==
  roll cmd : Inport
  roll model : Subsystem
  roll response : Outport
  roll rate : Outport  Port=2
  wires:
  roll model/2(roll rate) -> roll rate/1
  roll model/1(roll) -> roll response/1
  roll cmd/1 -> roll model/1(u_roll)

== system lab2_next_level/model/yaw model//controller ==
  yaw cmd : Inport
  yaw model : Subsystem
  yaw response : Outport
  yaw rate : Outport  Port=2
  wires:
  yaw model/2(yaw rate) -> yaw rate/1
  yaw cmd/1 -> yaw model/1(u_yaw)
  yaw model/1(yaw) -> yaw response/1

== system lab2_next_level/Platform/EnginePitch/PID2 ==
  In1 : Inport
  Derivative : Derivative
  Gain : Gain  Gain=2
  Gain1 : Gain  Gain=7.058823529e-07
  Gain2 : Gain  Gain=0.51875
  Gain3 : Gain
  Integrator : Integrator
  Sum1 : Sum  Inputs=|+++
  Out1 : Outport
  wires:
  Gain1/1 -> Integrator/1
  Gain3/1 -> Sum1/1
  Integrator/1 -> Sum1/2
  Gain/1 -> Gain3/1
  In1/1 -> Gain1/1, Gain/1, Gain2/1
  Derivative/1 -> Sum1/3
  Gain2/1 -> Derivative/1
  Sum1/1 -> Out1/1

== system lab2_next_level/Platform/EngineRoll/PID2 ==
  In1 : Inport
  Derivative : Derivative
  Gain : Gain  Gain=2
  Gain1 : Gain  Gain=7.058823529e-07
  Gain2 : Gain  Gain=0.51875
  Gain3 : Gain
  Integrator : Integrator
  Sum1 : Sum  Inputs=|+++
  Out1 : Outport
  wires:
  Gain1/1 -> Integrator/1
  Gain3/1 -> Sum1/1
  Integrator/1 -> Sum1/2
  Gain/1 -> Gain3/1
  In1/1 -> Gain1/1, Gain/1, Gain2/1
  Derivative/1 -> Sum1/3
  Gain2/1 -> Derivative/1
  Sum1/1 -> Out1/1

== system lab2_next_level/Platform/EngineYaw/PID2 ==
  In1 : Inport
  Derivative : Derivative
  Gain : Gain  Gain=2
  Gain1 : Gain  Gain=7.058823529e-07
  Gain2 : Gain  Gain=0.51875
  Gain3 : Gain
  Integrator : Integrator
  Sum1 : Sum  Inputs=|+++
  Out1 : Outport
  wires:
  Gain1/1 -> Integrator/1
  Gain3/1 -> Sum1/1
  Integrator/1 -> Sum1/2
  Gain/1 -> Gain3/1
  In1/1 -> Gain1/1, Gain/1, Gain2/1
  Derivative/1 -> Sum1/3
  Gain2/1 -> Derivative/1
  Sum1/1 -> Out1/1

== system lab2_next_level/model/pitch model//controller/pitch model ==
  u_pitch : Inport
  Demux : Demux
  State-Space : StateSpace  A=[0 1 0 0; 0 0 1600 0; 0 0 -15 0; 1 0 0 0]  B=[0;0;15;0]  C=[1 0 0 0; 0 1 0 0; 0 0 1 0; 0 0 0 1]  D=[0;0;0;0]
  Terminator_1 : Terminator
  Terminator_2 : Terminator
  pitch : Outport
  pitch rate : Outport  Port=2
  wires:
  Demux/4 -> Terminator_2/1
  Demux/3 -> Terminator_1/1
  u_pitch/1 -> State-Space/1
  Demux/2 -> pitch rate/1
  Demux/1 -> pitch/1
  State-Space/1 -> Demux/1

== system lab2_next_level/model/roll model//controller/roll model ==
  u_roll : Inport
  Demux : Demux
  State-Space : StateSpace  A=[0 1 0 0; 0 0 1600 0; 0 0 -15 0; 1 0 0 0]  B=[0;0;15;0]  C=[1 0 0 0; 0 1 0 0; 0 0 1 0; 0 0 0 1]  D=[0;0;0;0]
  Terminator_1 : Terminator
  Terminator_2 : Terminator
  roll : Outport
  roll rate : Outport  Port=2
  wires:
  Demux/4 -> Terminator_2/1
  Demux/3 -> Terminator_1/1
  u_roll/1 -> State-Space/1
  Demux/2 -> roll rate/1
  Demux/1 -> roll/1
  State-Space/1 -> Demux/1

== system lab2_next_level/model/yaw model//controller/yaw model ==
  u_yaw : Inport
  Integrator5 : Integrator
  Integrator6 : Integrator  LowerSaturationLimit=-0.5
  gain : Gain  Gain=4*4/0.032
  yaw : Outport
  yaw rate : Outport  Port=2
  wires:
  u_yaw/1 -> gain/1
  Integrator6/1 -> yaw/1
  gain/1 -> Integrator5/1
  Integrator5/1 -> yaw rate/1, Integrator6/1

== matlab function lab2_next_level/ControlSystem/MATLAB Function ==
  data: etalX input; etalY input; etalH input; curX input; curY input; curH input; counter input; error input; way input
function fcn(etalX,etalY,etalH,curX,curY,curH,counter,error,way)
%#codegen
coder.extrinsic('set_param');
coder.extrinsic('num2str');

[max,el] = size(way);

if abs(etalX-curX)<=error && abs(etalY-curY)<=error && abs(etalH-curH)<=error && counter<max,
    counter = counter + 1;
    set_param('lab2_next_level/ControlSystem/Constant1','Value',num2str(counter));
    set_param('lab2_next_level/ControlSystem/X','Value',num2str(way(counter,1)));
    set_param('lab2_next_level/ControlSystem/Y','Value',num2str(way(counter,2)));
    set_param('lab2_next_level/ControlSystem/H','Value',num2str(way(counter,3)));
end;

== matlab function lab2_next_level/AngularVelocitySensor/MATLAB Function ==
  data: roll input; pitch input; yaw input; x input; y input; z input; xs output; ys output; zs output
function [xs,ys,zs] = fromNavToAircraft(roll,pitch,yaw,x,y,z)
%#codegen
%from navigation to aircraft coordinate system

coder.extrinsic('rotationMatrix');

M = zeros(3,3,'double');
M = rotationMatrix(roll,pitch,yaw);
M = (M.')*[x;y;z];

xs = M(1);
ys = M(2);
zs = M(3);

== matlab function lab2_next_level/MATLAB Function1 ==
  data: roll input; pitch input; yaw input; x input; y input; z input; xs output; ys output; zs output
function [xs,ys,zs] = fromNavToAircraft(roll,pitch,yaw,x,y,z)
%#codegen
%from navigation to aircraft coordinate system
tr = [cos(pitch)*cos(yaw), -cos(roll)*sin(pitch)*cos(yaw)-sin(roll)*sin(yaw), sin(roll)*sin(pitch)*cos(yaw)-cos(roll)*sin(yaw);
      sin(pitch), cos(roll)*cos(pitch), -sin(roll)*cos(pitch);
      cos(pitch)*sin(yaw), -cos(roll)*sin(pitch)*sin(yaw)+sin(roll)*cos(yaw), sin(roll)*sin(pitch)*sin(yaw)+cos(roll)*cos(yaw)];
bx = [x;y;z];
ax = (tr.')*bx;

xs = ax(1);
ys = ax(2);
zs = ax(3);

== matlab function lab2_next_level/MATLAB Function2 ==
  data: roll input; pitch input; yaw input; x input; y input; z input; xs output; ys output; zs output
function [xs,ys,zs] = fromNavToAircraft(roll,pitch,yaw,x,y,z)
%#codegen
%from navigation to aircraft coordinate system
tr = [cos(pitch)*cos(yaw), -cos(roll)*sin(pitch)*cos(yaw)-sin(roll)*sin(yaw), sin(roll)*sin(pitch)*cos(yaw)-cos(roll)*sin(yaw);
      sin(pitch), cos(roll)*cos(pitch), -sin(roll)*cos(pitch);
      cos(pitch)*sin(yaw), -cos(roll)*sin(pitch)*sin(yaw)+sin(roll)*cos(yaw), sin(roll)*sin(pitch)*sin(yaw)+cos(roll)*cos(yaw)];
bx = [x;y;z];
ax = (tr.')*bx;

xs = ax(1);
ys = ax(2);
zs = ax(3);

== matlab function lab2_next_level/View/Visualisation ==
  data: x input; y input; z input; roll input; pitch input; yaw input; proll input; ppitch input; pyaw input; C input
function fcn(x,y,z,roll,pitch,yaw,proll,ppitch,pyaw,C)
%#codegen
coder.extrinsic('plot3')
coder.extrinsic('grid')
coder.extrinsic('axis')
coder.extrinsic('view')
coder.extrinsic('rotationMatrix');

if(C ~= 0)
    return
end

AXES = [100,0,0;0,100,0;0,0,100];

M = zeros(3,3,'double');
M = rotationMatrix(roll,pitch,yaw);
M = M*AXES;

MX = [x,M(1,1)+x;y,M(2,1)+y;z,M(3,1)+z];
MY = [x,M(1,2)+x;y,M(2,2)+y;z,M(3,2)+z];
MZ = [x,M(1,3)+x;y,M(2,3)+y;z,M(3,3)+z];

P = zeros(3,3,'double');
P = rotationMatrix(proll,ppitch,pyaw);
P = P*AXES;

PX = [x,P(1,1)+x;y,P(2,1)+y;z,P(3,1)+z];
PY = [x,P(1,2)+x;y,P(2,2)+y;z,P(3,2)+z];
PZ = [x,P(1,3)+x;y,P(2,3)+y;z,P(3,3)+z];

[az, el] = view;
plot3(x,y,z, 'or',MX(1,:),MX(2,:),MX(3,:), '-r',MY(1,:),MY(2,:),MY(3,:), '-g',MZ(1,:),MZ(2,:),MZ(3,:), '-b',PX(1,:),PX(2,:),PX(3,:), '--m',PY(1,:),PY(2,:),PY(3,:), '--k',PZ(1,:),PZ(2,:),PZ(3,:), '--c',[x+50,x+50,x-50,x-50,x+50],[y+50,y-50,y-50,y+50,y+50],[z,z,z,z,z]);
axis([-1000 1000 -1000 1000 0 500])
grid on
view([az, el]);


end

== matlab function lab2_next_level/model2/accel ==
  data: P input; a_x output; angles input; a_y output; a_z output
function [a_x, a_y, a_z] = fcn(P, angles)

roll = angles(1);
pitch = angles(2);
yaw = angles(3);

C_x = [1,0,0;
       0, cos(roll), sin(roll);
       0, -sin(roll), cos(roll)];
C_y = [cos(pitch),0,-sin(pitch);
       0, 1, 0;
       sin(pitch), 0, cos(pitch)];
C_z = [cos(yaw),sin(yaw),0;
       -sin(yaw), cos(yaw), 0;
       0, 0, 1];
   
C = C_z*C_x*C_y;

proectP = C*[0;0;1];

P_sum = sum(P);


k_x = 0.9;
k_y = 0.9;
k_z = 0.9;

m = 10;
g = 9.8;

a_x = proectP(1)*P_sum * k_x / m;

a_y = proectP(2)*P_sum * k_y / m;

a_z = proectP(3)*P_sum * k_z / m - g;

== matlab function lab2_next_level/model2/angle_accel ==
  data: P input; ddroll output; ddpitch output; ddyaw output
function [ddroll, ddpitch, ddyaw] = fcn(P)

%distance between oneside engine
h = 0.5;

Jx = 1;
Jy = 1;
Jz = 1;

M_x = (P(1)-P(2)+P(3)-P(4))*h/Jx;
M_y = (P(1)+P(2)-P(3)-P(4))*h/Jy;
k=0.5;
M_z = (P(1)+P(4)-P(2)-P(3))*h*k/Jz;

k_roll = 0.8;
k_pitch = 0.8;
k_yaw = 0.8;


ddroll = M_x * k_roll;
ddpitch = M_y * k_pitch;
ddyaw = M_z * k_yaw;

== matlab function lab2_next_level/ControlSystemOrigin/MATLAB Function ==
  data: etalX input; etalY input; etalH input; curX input; curY input; curH input; counter input; error input; way input
function fcn(etalX,etalY,etalH,curX,curY,curH,counter,error,way)
%#codegen
coder.extrinsic('set_param');
coder.extrinsic('num2str');

[max,el] = size(way);

if abs(etalX-curX)<=error && abs(etalY-curY)<=error && abs(etalH-curH)<=error && counter<max,
    counter = counter + 1;
    set_param('lab2_next_level/ControlSystem/Constant1','Value',num2str(counter));
    set_param('lab2_next_level/ControlSystem/X','Value',num2str(way(counter,1)));
    set_param('lab2_next_level/ControlSystem/Y','Value',num2str(way(counter,2)));
    set_param('lab2_next_level/ControlSystem/H','Value',num2str(way(counter,3)));
end;

== matlab function lab2_next_level/Platform/MATLAB Function ==
  data: roll input; pitch input; yaw input; x input; y input; z input; xs output; ys output; zs output
function [xs,ys,zs] = fromAircraftToPlatform(roll,pitch,yaw,x,y,z)
%#codegen
%from navigation to aircraft coordinate system

coder.extrinsic('rotationMatrix');
roll = 0;pitch= 0;

cr = cos(roll);     sr = sin(roll); 
cp = cos(pitch);    sp = sin(pitch);
cy = cos(yaw);      sy = sin(yaw);

CY = [cp,0,-sp;0,1,0;sp,0,cp];
CX = [1,0,0;0,cr,sr;0,-sr,cr];
CZ = [cy,sy,0;-sy,cy,0;0,0,1];

M = CZ*[x;y;z];

xs = M(1);
ys = M(2);
zs = M(3);

== matlab function lab2_next_level/AngularVelocitySensor/MATLAB Function1 ==
  data: roll input; pitch input; yaw input; x input; y input; z input; xs output; ys output; zs output
function [xs,ys,zs] = fromNavToAircraft(roll,pitch,yaw,x,y,z)
%#codegen
%from navigation to aircraft coordinate system

coder.extrinsic('rotationMatrix');

M = zeros(3,3,'double');
M = rotationMatrix(roll,pitch,yaw);
M = M*[x;y;z];

xs = M(1);
ys = M(2);
zs = M(3);

== matlab function lab2_next_level/Platform/MATLAB Function1 ==
  data: roll input; pitch input; yaw input; x input; y input; z input; xs output; ys output; zs output
function [xs,ys,zs] = fromAircraftToPlatform(roll,pitch,yaw,x,y,z)
%#codegen
%from navigation to aircraft coordinate system

coder.extrinsic('rotationMatrix');
roll = 0;pitch= 0;

cr = cos(roll);     sr = sin(roll); 
cp = cos(pitch);    sp = sin(pitch);
cy = cos(yaw);      sy = sin(yaw);

CY = [cp,0,-sp;0,1,0;sp,0,cp];
CX = [1,0,0;0,cr,sr;0,-sr,cr];
CZ = [cy,sy,0;-sy,cy,0;0,0,1];

M = CZ'*[x;y;z];

xs = M(1);
ys = M(2);
zs = M(3);
